simulink library "Lib_PF_ImpedanceAC_TMATS"  (R2017a)
settings: Solver=ode45  StartTime=0.0  StopTime=10.0  RelTol=1e-3  EnableMultiTasking=on
Description:
  | Thomas Modules
settings Model: Creator=jwchapm2  LastModifiedBy=glthoma1
settings DataIOCC: LimitDataPoints=on  SaveFormat=Array
settings OptimizationCC: ExpressionDepthLimit=2147483647  LifeSpan=inf
settings DebuggingCC: UnderspecifiedInitializationDetection=Classic  MergeDetectMultiDrivingBlocksExec=none  SolverPrmCheckMsg=warning  StateNameClashWarn=warning  SFUnexpectedBacktrackingDiag=warning  SFNoUnconditionalDefaultTransitionDiag=warning  SFExecutionAtInitializationDiag=none
settings HardwareCC: ProdBitPerPointer=32  ProdBitPerSizeT=32  ProdBitPerPtrDiffT=32  ProdLargestAtomicFloat=None  ProdIntDivRoundTo=Undefined  ProdEndianess=Unspecified  ProdWordSize=32  ProdHWDeviceType=32-bit Generic
settings ModelReferenceCC: PropagateSignalLabelsOutOfModel=off
settings GRTTargetCC: TargetLangStandard=C89/C90 (ANSI)  GeneratePreprocessorConditionals=Disable all
settings ConfigComp: CovMetricSettings=dw  CovHtmlReporting=on  CovSaveCumulativeToWorkspaceVar=on  CovSaveSingleToWorkspaceVar=on  CovExternalEMLEnable=off

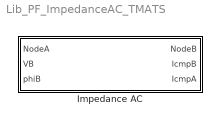
== system Lib_PF_ImpedanceAC_TMATS ==
  Impedance AC : Subsystem  mask{R_M=100, X_M=0.015}
      mask prompts: R_M "R_M - Resistance"; X_M "X_M - Reactance"
      mask Display:
      | fprintf('R + jX\n %g + j%g',R_M, X_M)
      | port_label('input',1,'VA')
      | port_label('input',2,'VBg')
      | port_label('input',3,'phiBg')
      | port_label('output',1,'VB')
      | port_label('output',2,'IcB')
      | port_label('output',3,'IcA')

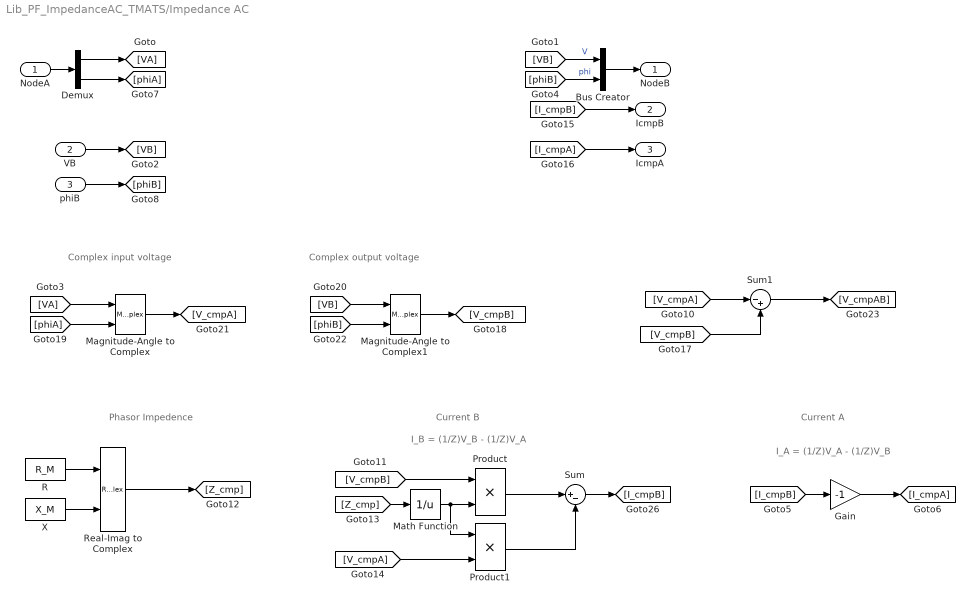
== system Lib_PF_ImpedanceAC_TMATS/Impedance AC ==
  note: Complex output voltage
  note: Complex input voltage
  note: Phasor Impedence
  note: Current B
  note: Current A
  note: I_B = (1/Z)V_B - (1/Z)V_A
  note: I_A = (1/Z)V_A - (1/Z)V_B
  NodeA : Inport
  VB : Inport  Port=2
  phiB : Inport  Port=3
  Bus Creator : BusCreator  Inputs=2
  Demux : Demux  Outputs=2
  Gain : Gain  Gain=-1
  Magnitude-Angle to Complex : MagnitudeAngleToComplex
  Magnitude-Angle to Complex1 : MagnitudeAngleToComplex
  Math Function : Math  Operator=reciprocal  SaturateOnIntegerOverflow=on
  Product : Product
  Product1 : Product
  R : Constant  Value=R_M
  Real-Imag to Complex : RealImagToComplex
  Sum : Sum  Inputs=|+-
  Sum1 : Sum  Inputs=|-+
  X : Constant  Value=X_M
  NodeB : Outport
  IcmpB : Outport  Port=2
  IcmpA : Outport  Port=3
  wires:
  Demux/1 -> [VA]
  [phiB] -> Bus Creator/2  "phi"
  [I_cmpB] -> IcmpB/1
  phiB/1 -> [phiB]
  Demux/2 -> [phiA]
  NodeA/1 -> Demux/1
  VB/1 -> [VB]
  [VB] -> Bus Creator/1  "V"
  Bus Creator/1 -> NodeB/1
  [VA] -> Magnitude-Angle to Complex/1
  [phiA] -> Magnitude-Angle to Complex/2
  Magnitude-Angle to Complex/1 -> [V_cmpA]
  [VB] -> Magnitude-Angle to Complex1/1
  Magnitude-Angle to Complex1/1 -> [V_cmpB]
  [phiB] -> Magnitude-Angle to Complex1/2
  R/1 -> Real-Imag to Complex/1
  X/1 -> Real-Imag to Complex/2
  Real-Imag to Complex/1 -> [Z_cmp]
  [V_cmpB] -> Product/1
  [Z_cmp] -> Math Function/1
  Sum/1 -> [I_cmpB]
  Math Function/1 -> Product1/1, Product/2
  [I_cmpA] -> IcmpA/1
  [V_cmpA] -> Product1/2
  Product1/1 -> Sum/2
  Product/1 -> Sum/1
  [I_cmpB] -> Gain/1
  Gain/1 -> [I_cmpA]
  [V_cmpA] -> Sum1/1
  [V_cmpB] -> Sum1/2
  Sum1/1 -> [V_cmpAB]
